simulink model "m040_NewtonCoolingLaw"  (R2022a)
settings: Solver=VariableStepAuto  StartTime=0.0  StopTime=50  RelTol=1e-3
settings Model: Creator=Admin  LastModifiedBy=Admin

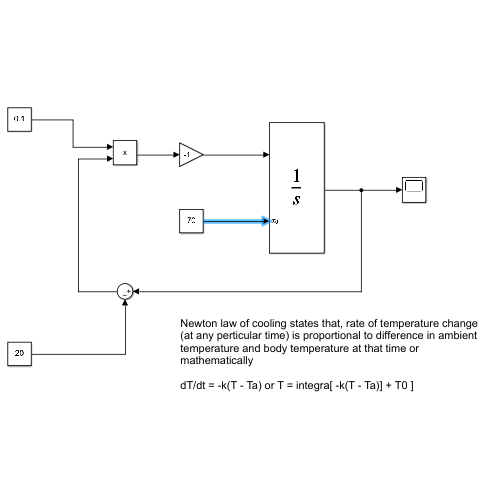
[thumbnail: Simulink's stored preview of the top-level diagram]
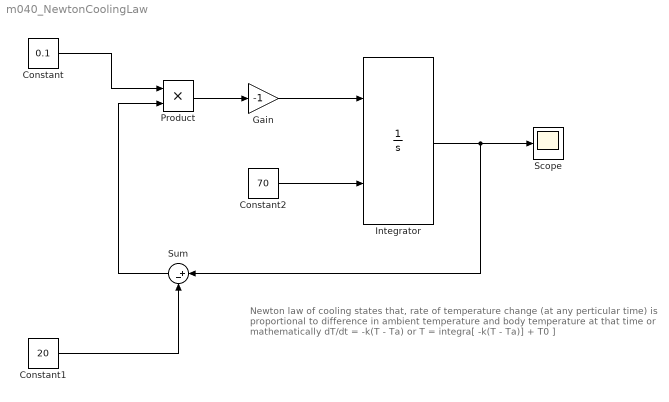
== system m040_NewtonCoolingLaw ==
  note: Newton law of cooling states that, rate of temperature change (at any perticular time) is proportional to difference in ambient temperature and body temperature at that time or mathematically
      |
      | dT/dt = -k(T - Ta) or T = integra[ -k(T - Ta)] + T0 ]
  Constant : Constant  Value=0.1
  Constant1 : Constant  Value=20
  Constant2 : Constant  Value=70
  Gain : Gain  Gain=-1
  Integrator : Integrator  InitialConditionSource=external
  Product : Product
  Scope : Scope
  Sum : Sum  Inputs=|+-
  wires:
  Constant/1 -> Product/1
  Constant1/1 -> Sum/2
  Integrator/1 -> Sum/1, Scope/1
  Constant2/1 -> Integrator/2
  Gain/1 -> Integrator/1
  Product/1 -> Gain/1
  Sum/1 -> Product/2
